simulink library "efiLib"  (R2018a)
settings: Solver=VariableStepAuto  StartTime=0.0  StopTime=10.0  RelTol=1e-3
settings Model: Creator=SIMONE  LastModifiedBy=SIMONE

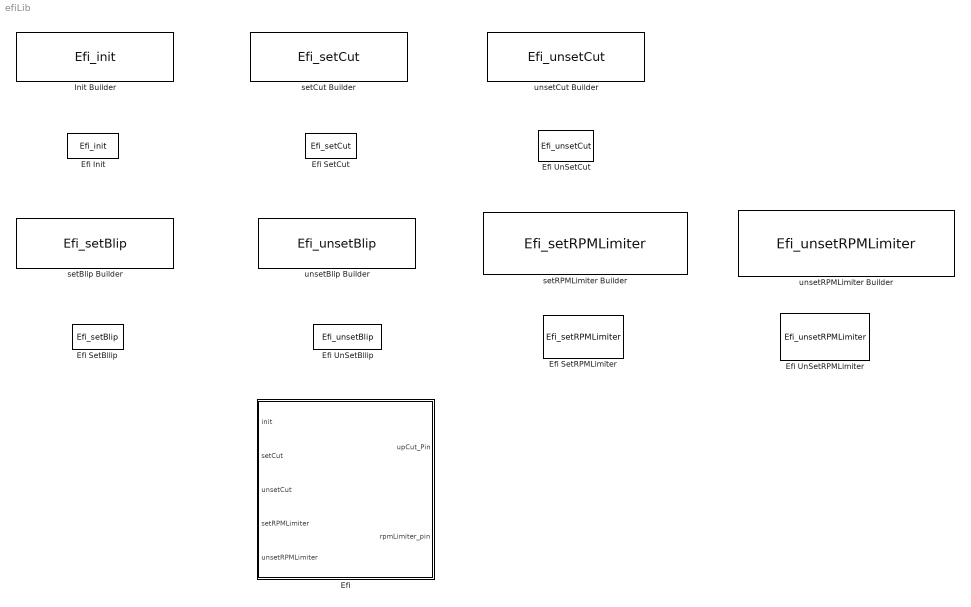
== system efiLib ==
  Efi : Subsystem
  Efi Init : S-Function  FunctionName=Efi_init  SFunctionDeploymentMode=off  EnableBusSupport=off
  Efi SetBllip : S-Function  FunctionName=Efi_setBlip  SFunctionDeploymentMode=off  EnableBusSupport=off
  Efi SetCut : S-Function  FunctionName=Efi_setCut  SFunctionDeploymentMode=off  EnableBusSupport=off
  Efi SetRPMLimiter : S-Function  FunctionName=Efi_setRPMLimiter  SFunctionDeploymentMode=off  EnableBusSupport=off
  Efi UnSetBllip : S-Function  FunctionName=Efi_unsetBlip  SFunctionDeploymentMode=off  EnableBusSupport=off
  Efi UnSetCut : S-Function  FunctionName=Efi_unsetCut  SFunctionDeploymentMode=off  EnableBusSupport=off
  Efi UnSetRPMLimiter : S-Function  FunctionName=Efi_unsetRPMLimiter  SFunctionDeploymentMode=off  EnableBusSupport=off
  Init Builder : S-Function  InitFcn=try, set_param(gcb,'FunctionName','Efi_init'), end  FunctionName=Efi_init  SFunctionModules=Efi_init_wrapper  SFunctionDeploymentMode=off  EnableBusSupport=off  mask(S-Function Builder){}
      mask help: Simulink:masks:SFunctionBuilder_MD
      mask init:
      | val = [[.9  0.75 0.75 1 1 .9 .9 1]',[1 1 0.75 0.75 .9 .9 1 .9]'];try , sys = get_param(gcb,'SfunBuilderFcnName');if isempty(sys), sys = get_param(gcb,'FunctionName'); end,catch, sys = get_param(gcb,'FunctionName'); end
      settings: CopyFcn=set_param(gcbh,'LinkStatus','none')  PreSaveFcn=try, set_param(gcb,'FunctionName','Efi_init'), end  OpenFcn=sfunctionwizard(gcbh)
      mask Display:
      | plot(val(:,1),val(:,2))
      | disp(sys)
  setBlip Builder : S-Function  InitFcn=try, set_param(gcb,'FunctionName','Efi_setBlip'), end  FunctionName=Efi_setBlip  SFunctionModules=Efi_setBlip_wrapper  SFunctionDeploymentMode=off  EnableBusSupport=off  mask(S-Function Builder){}
      mask help: Simulink:masks:SFunctionBuilder_MD
      mask init: same as efiLib/Init Builder
      settings: CopyFcn=set_param(gcbh,'LinkStatus','none')  PreSaveFcn=try, set_param(gcb,'FunctionName','Efi_setBlip'), end  OpenFcn=sfunctionwizard(gcbh)
      mask Display: plot(val(:,1),val(:,2)),disp(sys), port_label('output',1,'downCut_pin')
  setCut Builder : S-Function  InitFcn=try, set_param(gcb,'FunctionName','Efi_setCut'), end  FunctionName=Efi_setCut  SFunctionModules=Efi_setCut_wrapper  SFunctionDeploymentMode=off  EnableBusSupport=off  mask(S-Function Builder){}
      mask help: Simulink:masks:SFunctionBuilder_MD
      mask init: same as efiLib/Init Builder
      settings: CopyFcn=set_param(gcbh,'LinkStatus','none')  PreSaveFcn=try, set_param(gcb,'FunctionName','Efi_setCut'), end  OpenFcn=sfunctionwizard(gcbh)
      mask Display: plot(val(:,1),val(:,2)),disp(sys), port_label('output',1,'upCut_pin')
  setRPMLimiter Builder : S-Function  InitFcn=try, set_param(gcb,'FunctionName','Efi_setRPMLimiter'), end  FunctionName=Efi_setRPMLimiter  SFunctionModules=Efi_setRPMLimiter_wrapper  SFunctionDeploymentMode=off  EnableBusSupport=off  mask(S-Function Builder){}
      mask help: Simulink:masks:SFunctionBuilder_MD
      mask init: same as efiLib/Init Builder
      settings: CopyFcn=set_param(gcbh,'LinkStatus','none')  PreSaveFcn=try, set_param(gcb,'FunctionName','Efi_setRPMLimiter'), end  OpenFcn=sfunctionwizard(gcbh)
      mask Display: plot(val(:,1),val(:,2)),disp(sys), port_label('output',1,'rpmLimiter_pin')
  unsetBlip Builder : S-Function  InitFcn=try, set_param(gcb,'FunctionName','Efi_unsetBlip'), end  FunctionName=Efi_unsetBlip  SFunctionModules=Efi_unsetBlip_wrapper  SFunctionDeploymentMode=off  EnableBusSupport=off  mask(S-Function Builder){}
      mask help: Simulink:masks:SFunctionBuilder_MD
      mask init: same as efiLib/Init Builder
      settings: CopyFcn=set_param(gcbh,'LinkStatus','none')  PreSaveFcn=try, set_param(gcb,'FunctionName','Efi_unsetBlip'), end  OpenFcn=sfunctionwizard(gcbh)
      mask Display: plot(val(:,1),val(:,2)),disp(sys), port_label('output',1,'downCut_pin')
  unsetCut Builder : S-Function  InitFcn=try, set_param(gcb,'FunctionName','Efi_unsetCut'), end  FunctionName=Efi_unsetCut  SFunctionModules=Efi_unsetCut_wrapper  SFunctionDeploymentMode=off  EnableBusSupport=off  mask(S-Function Builder){}
      mask help: Simulink:masks:SFunctionBuilder_MD
      mask init: same as efiLib/Init Builder
      settings: CopyFcn=set_param(gcbh,'LinkStatus','none')  PreSaveFcn=try, set_param(gcb,'FunctionName','Efi_unsetCut'), end  OpenFcn=sfunctionwizard(gcbh)
      mask Display: plot(val(:,1),val(:,2)),disp(sys), port_label('output',1,'upCut_pin')
  unsetRPMLimiter Builder : S-Function  InitFcn=try, set_param(gcb,'FunctionName','Efi_unsetRPMLimiter'), end  FunctionName=Efi_unsetRPMLimiter  SFunctionModules=Efi_unsetRPMLimiter_wrapper  SFunctionDeploymentMode=off  EnableBusSupport=off  mask(S-Function Builder){}
      mask help: Simulink:masks:SFunctionBuilder_MD
      mask init: same as efiLib/Init Builder
      settings: CopyFcn=set_param(gcbh,'LinkStatus','none')  PreSaveFcn=try, set_param(gcb,'FunctionName','Efi_unsetRPMLimiter'), end  OpenFcn=sfunctionwizard(gcbh)
      mask Display: plot(val(:,1),val(:,2)),disp(sys), port_label('output',1,'rpmLimiter_pin')

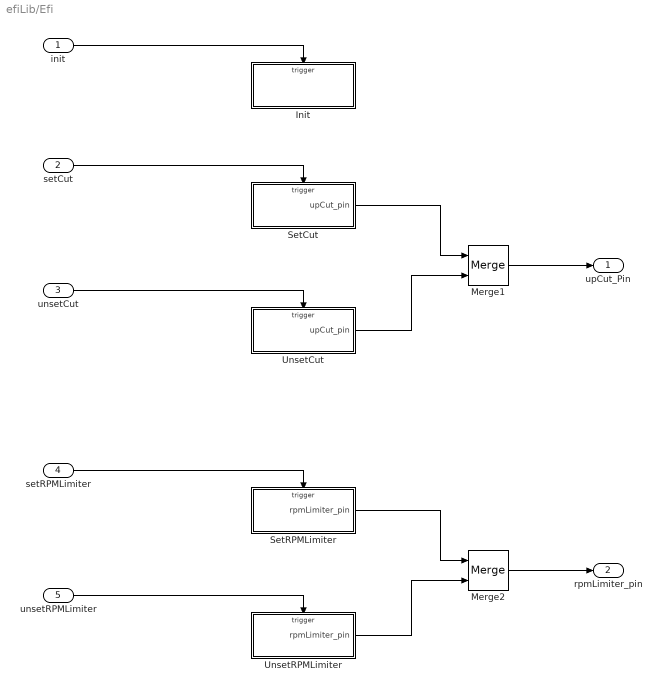
== system efiLib/Efi ==
  init : Inport
  setCut : Inport  Port=2
  unsetCut : Inport  Port=3
  setRPMLimiter : Inport  Port=4
  unsetRPMLimiter : Inport  Port=5
  Init : Subsystem  TreatAsAtomicUnit=on
  Merge1 : Merge
  Merge2 : Merge
  SetCut : Subsystem  TreatAsAtomicUnit=on
  SetRPMLimiter : Subsystem  AncestorBlock=efiLib/Efi/SetCut  TreatAsAtomicUnit=on
  UnsetCut : Subsystem  TreatAsAtomicUnit=on
  UnsetRPMLimiter : Subsystem  AncestorBlock=efiLib/Efi/UnsetCut  TreatAsAtomicUnit=on
  upCut_Pin : Outport
  rpmLimiter_pin : Outport  Port=2
  wires:
  init/1 -> Init/Trigger
  setCut/1 -> SetCut/Trigger
  unsetCut/1 -> UnsetCut/Trigger
  UnsetCut/1(upCut_pin) -> Merge1/2
  SetCut/1(upCut_pin) -> Merge1/1
  Merge1/1 -> upCut_Pin/1
  UnsetRPMLimiter/1(rpmLimiter_pin) -> Merge2/2
  setRPMLimiter/1 -> SetRPMLimiter/Trigger
  Merge2/1 -> rpmLimiter_pin/1
  SetRPMLimiter/1(rpmLimiter_pin) -> Merge2/1
  unsetRPMLimiter/1 -> UnsetRPMLimiter/Trigger

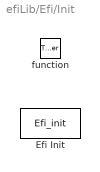
== system efiLib/Efi/Init ==
  function : TriggerPort  TriggerType=function-call  VariantControl=Variant
  Efi Init : S-Function  FunctionName=Efi_init  SFunctionDeploymentMode=off  EnableBusSupport=off

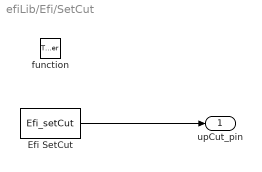
== system efiLib/Efi/SetCut ==
  function : TriggerPort  TriggerType=function-call  VariantControl=Variant
  Efi SetCut : S-Function  FunctionName=Efi_setCut  SFunctionDeploymentMode=off  EnableBusSupport=off
  upCut_pin : Outport
  wires:
  Efi SetCut/1 -> upCut_pin/1

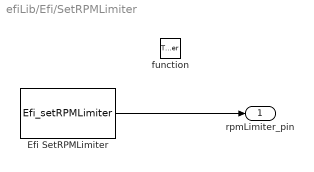
== system efiLib/Efi/SetRPMLimiter ==
  function : TriggerPort  TriggerType=function-call  VariantControl=Variant
  Efi SetRPMLimiter : S-Function  FunctionName=Efi_setRPMLimiter  SFunctionDeploymentMode=off  EnableBusSupport=off
  rpmLimiter_pin : Outport
  wires:
  Efi SetRPMLimiter/1 -> rpmLimiter_pin/1

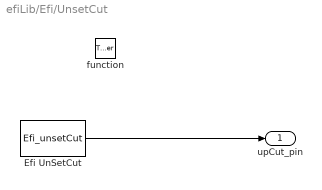
== system efiLib/Efi/UnsetCut ==
  function : TriggerPort  TriggerType=function-call  VariantControl=Variant
  Efi UnSetCut : S-Function  FunctionName=Efi_unsetCut  SFunctionDeploymentMode=off  EnableBusSupport=off
  upCut_pin : Outport
  wires:
  Efi UnSetCut/1 -> upCut_pin/1

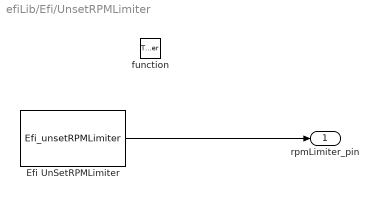
== system efiLib/Efi/UnsetRPMLimiter ==
  function : TriggerPort  TriggerType=function-call  VariantControl=Variant
  Efi UnSetRPMLimiter : S-Function  FunctionName=Efi_unsetRPMLimiter  SFunctionDeploymentMode=off  EnableBusSupport=off
  rpmLimiter_pin : Outport
  wires:
  Efi UnSetRPMLimiter/1 -> rpmLimiter_pin/1
